simulink model "Disturbancce_Observe"  (R2014b)
settings: Solver=ode45  StartTime=0.0  StopTime=10.0  RelTol=1e-3
libraries: simulink x1
settings Model: Creator=wangsp1  LastModifiedBy=wangsp1

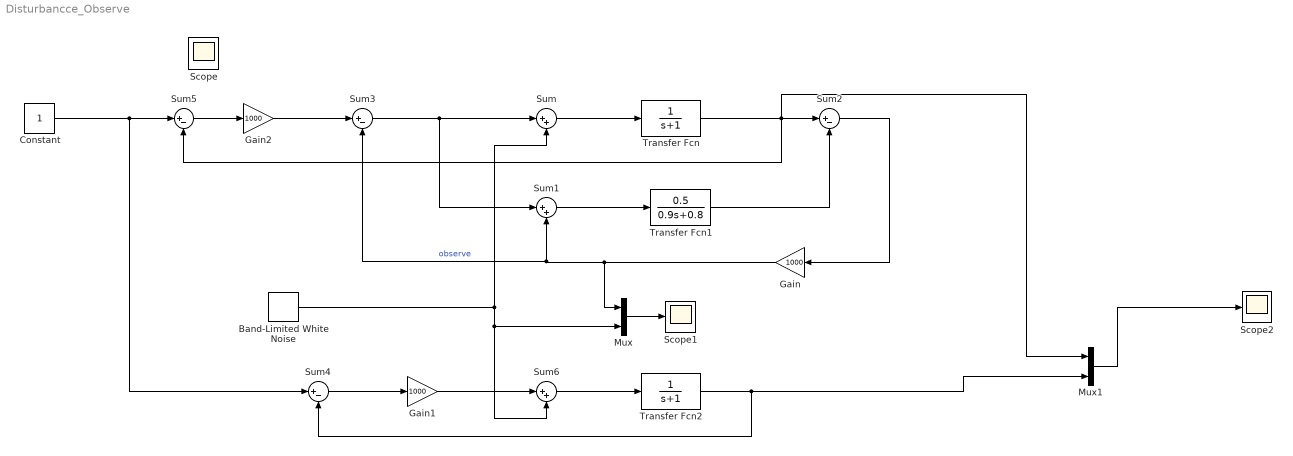
== system Disturbancce_Observe ==
  Band-Limited White Noise : simulink/Sources/Band-Limited White Noise  Cov=[10.1]  Ts=0.01  seed=[23341]
  Constant : Constant
  Gain : Gain  Gain=1000
  Gain1 : Gain  Gain=1000
  Gain2 : Gain  Gain=1000
  Mux : Mux  Inputs=2
  Mux1 : Mux  Inputs=2
  Scope1 : Scope
  Scope2 : Scope
      settings: SaveName=ScopeData2
  Sum : Sum  Inputs=|++
  Sum1 : Sum  Inputs=|++
  Sum{2..5} (4 alike) : Sum  Inputs=|+-
  Sum6 : Sum  Inputs=|++
  Transfer Fcn : TransferFcn  Denominator=[1 1]
  Transfer Fcn1 : TransferFcn  Numerator=[0.5]  Denominator=[0.9 0.8]
  Transfer Fcn2 : TransferFcn  Denominator=[1 1]
  Scope : Scope
  wires:
  Sum/1 -> Transfer Fcn/1
  Sum1/1 -> Transfer Fcn1/1
  Transfer Fcn/1 -> Sum5/2, Mux1/1, Sum2/1
  Transfer Fcn1/1 -> Sum2/2
  Sum2/1 -> Gain/1
  Band-Limited White Noise/1 -> Mux/2, Sum6/2, Sum/2
  Gain/1 -> Mux/1, Sum3/2, Sum1/2  "observe"
  Mux/1 -> Scope1/1
  Constant/1 -> Sum5/1, Sum4/1
  Sum3/1 -> Sum1/1, Sum/1
  Sum4/1 -> Gain1/1
  Transfer Fcn2/1 -> Mux1/2, Sum4/2
  Mux1/1 -> Scope2/1
  Sum5/1 -> Gain2/1
  Gain2/1 -> Sum3/1
  Gain1/1 -> Sum6/1
  Sum6/1 -> Transfer Fcn2/1
